simulink model "pdl_linear_hw4hybrid"  (R2017a)
settings: Solver=FixedStepAuto  StartTime=0.0  StopTime=duration  FixedStep=Ts  RelTol=1e-3
values from neighbouring files (symbols this model uses):
  A_a = [A E*Cw; zeros(2,4) Aw]    [pendulum_hw4linear.m]
  B_a = [B; zeros(2,1)]    [pendulum_hw4linear.m]
  C_a = [C zeros(2,2)]    [pendulum_hw4linear.m]
  E_a = [zeros(4,2); Bw]    [pendulum_hw4linear.m]
  f_p = 1e-4    (= 0.0001)    [pendulum_hw4linear.m]
  m_p = 1e-7    (= 1e-07)    [pendulum_hw4linear.m]
  Q_k1 = diag([10.00001 10.001])    [pendulum_hw4linear.m]
  Q_k2 = diag([10.00007 9.997])    [pendulum_hw4linear.m]
  Q_k3 = diag([10.0000905 9.995])    [pendulum_hw4linear.m]
  Q_k4 = diag([10.000101 9.9935])    [pendulum_hw4linear.m]
  R_k1 = 1e-5*diag([1 1])    [pendulum_hw4linear.m]
  R_k2 = 1e-5*diag([1 1])    [pendulum_hw4linear.m]
  R_k3 = 1e-5*diag([1 1])    [pendulum_hw4linear.m]
  R_k4 = 1e-5*diag([1 1])    [pendulum_hw4linear.m]
  Ts = 0.001    [pendulum_hw4linear.m]
  w_p = 10    [pendulum_hw4linear.m]
  X_0 = [0;0*pi/180;0;0;0;0]    [pendulum_hw4linear.m]
undefined symbols (not defined in the file or in its folder): Delta, Gamma, LC1_D, LC2_D, LC3_D, LC4_D, Phi
libraries: simulink x3
settings Model: Creator=Salmon  LastModifiedBy=Salmon

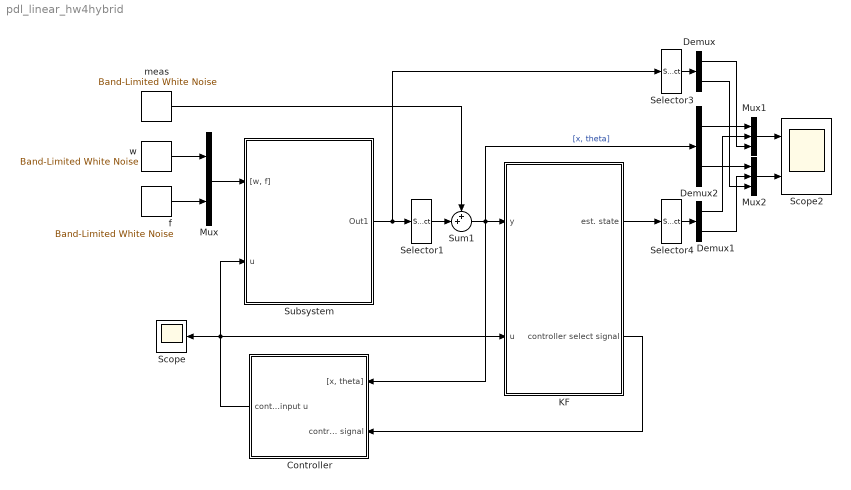
== system pdl_linear_hw4hybrid ==
  Controller : Subsystem
  Demux : Demux  Outputs=2
  Demux1 : Demux  Outputs=2
  Demux2 : Demux  Outputs=2
  KF : Subsystem
  Mux : Mux  Inputs=2
  Mux1 : Mux  Inputs=3
  Mux2 : Mux  Inputs=3
  Scope : Scope
  Scope2 : Scope  NumInputPorts=2
  Selector1 : Selector  InputPortWidth=6  IndexOptions=Index vector (dialog)  Indices=[1 2]  OutputSizes=1
  Selector3 : Selector  InputPortWidth=6  IndexOptions=Index vector (dialog)  Indices=[1 2]  OutputSizes=1
  Selector4 : Selector  InputPortWidth=6  IndexOptions=Index vector (dialog)  Indices=[1 2]  OutputSizes=1
  Subsystem : Subsystem
  Sum1 : Sum  Inputs=++|
  f : simulink/Sources/Band-Limited White Noise  Cov=[f_p]  Ts=Ts  seed=[23341]
  meas : simulink/Sources/Band-Limited White Noise  Cov=[m_p,m_p]  Ts=Ts  seed=[123,23341]
  w : simulink/Sources/Band-Limited White Noise  Cov=[w_p]  Ts=Ts  seed=[23341]
  wires:
  w/1 -> Mux/1
  f/1 -> Mux/2
  Mux/1 -> Subsystem/1("[w, f]")
  Subsystem/1(Out1) -> Selector1/1, Selector3/1
  Demux/1 -> Mux1/3
  Demux/2 -> Mux2/3
  Selector1/1 -> Sum1/2
  Demux1/1 -> Mux1/2
  KF/2(controller select signal) -> Controller/2(controller select signal)
  Demux1/2 -> Mux2/2
  meas/1 -> Sum1/1
  Demux2/1 -> Mux1/1
  Demux2/2 -> Mux2/1
  Mux1/1 -> Scope2/1
  Mux2/1 -> Scope2/2
  Sum1/1 -> Controller/1("[x, theta]"), KF/1(y), Demux2/1  "[x, theta]"
  Selector3/1 -> Demux/1
  Selector4/1 -> Demux1/1
  Controller/1(control input u) -> Subsystem/2(u), KF/2(u), Scope/1
  KF/1(est. state) -> Selector4/1

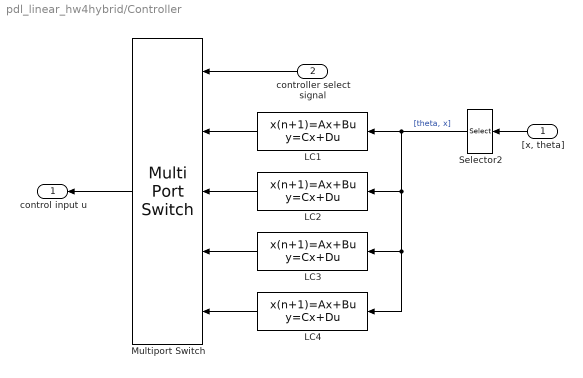
== system pdl_linear_hw4hybrid/Controller ==
  "[x, theta]" : Inport
  controller select signal : Inport  Port=2
  LC1 : DiscreteStateSpace  A=LC1_D.A  B=LC1_D.B  C=LC1_D.C  D=LC1_D.D  SampleTime=Ts
  LC2 : DiscreteStateSpace  A=LC2_D.A  B=LC2_D.B  C=LC2_D.C  D=LC2_D.D  SampleTime=Ts
  LC3 : DiscreteStateSpace  A=LC3_D.A  B=LC3_D.B  C=LC3_D.C  D=LC3_D.D  SampleTime=Ts
  LC4 : DiscreteStateSpace  A=LC4_D.A  B=LC4_D.B  C=LC4_D.C  D=LC4_D.D  SampleTime=Ts
  Multiport Switch : MultiPortSwitch  Inputs=4  DiagnosticForDefault=None
  Selector2 : Selector  InputPortWidth=2  IndexOptions=Index vector (dialog)  Indices=[2 1]  OutputSizes=1
  control input u : Outport
  wires:
  LC4/1 -> Multiport Switch/5
  controller select signal/1 -> Multiport Switch/1
  LC3/1 -> Multiport Switch/4
  LC2/1 -> Multiport Switch/3
  LC1/1 -> Multiport Switch/2
  Selector2/1 -> LC4/1, LC3/1, LC2/1, LC1/1  "[theta, x]"
  Multiport Switch/1 -> control input u/1
  "[x, theta]"/1 -> Selector2/1

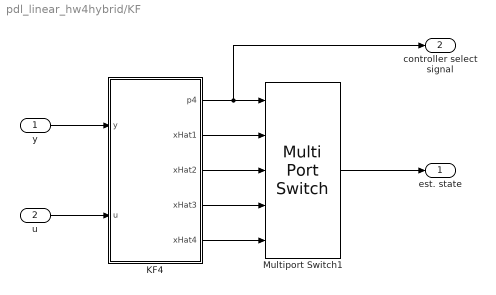
== system pdl_linear_hw4hybrid/KF ==
  y : Inport
  u : Inport  Port=2
  KF4 : Subsystem
  Multiport Switch1 : MultiPortSwitch  Inputs=4  DiagnosticForDefault=None
  est. state : Outport
  controller select signal : Outport  Port=2
  wires:
  u/1 -> KF4/2(u)
  Multiport Switch1/1 -> est. state/1
  y/1 -> KF4/1(y)
  KF4/5("xHat4 ") -> Multiport Switch1/5
  KF4/4(xHat3) -> Multiport Switch1/4
  KF4/3(xHat2) -> Multiport Switch1/3
  KF4/2(xHat1) -> Multiport Switch1/2
  KF4/1(p4) -> controller select signal/1, Multiport Switch1/1

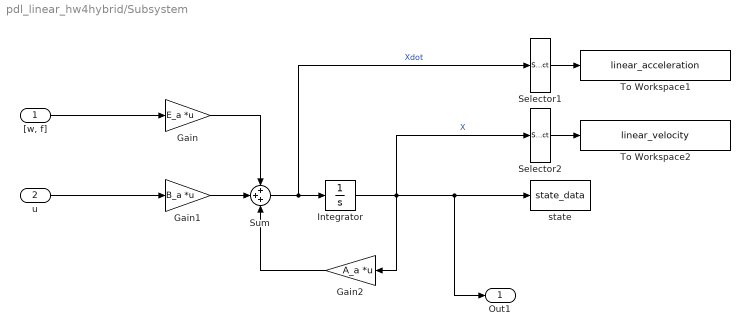
== system pdl_linear_hw4hybrid/Subsystem ==
  "[w, f]" : Inport
  u : Inport  Port=2
  Gain : Gain  Gain=E_a  Multiplication=Matrix(K*u)
  Gain1 : Gain  Gain=B_a  Multiplication=Matrix(K*u)
  Gain2 : Gain  Gain=A_a  Multiplication=Matrix(K*u)
  Integrator : Integrator  InitialCondition=X_0
  Selector1 : Selector  InputPortWidth=6  IndexOptions=Index vector (dialog)  Indices=[3]  OutputSizes=1
  Selector2 : Selector  InputPortWidth=6  IndexOptions=Index vector (dialog)  Indices=[3]  OutputSizes=1
  Sum : Sum  Inputs=+++
  To Workspace1 : ToWorkspace  VariableName=linear_acceleration  SaveFormat=Structure With Time  SampleTime=-1
  To Workspace2 : ToWorkspace  VariableName=linear_velocity  SaveFormat=Structure With Time  SampleTime=-1
  state : ToWorkspace  VariableName=state_data  SaveFormat=Structure With Time  SampleTime=Ts
  Out1 : Outport
  wires:
  "[w, f]"/1 -> Gain/1
  Gain/1 -> Sum/1
  Gain1/1 -> Sum/2
  Selector2/1 -> To Workspace2/1
  Selector1/1 -> To Workspace1/1
  Gain2/1 -> Sum/3
  u/1 -> Gain1/1
  Integrator/1 -> Gain2/1, Selector2/1, Out1/1, state/1  "X"
  Sum/1 -> Integrator/1, Selector1/1  "Xdot"

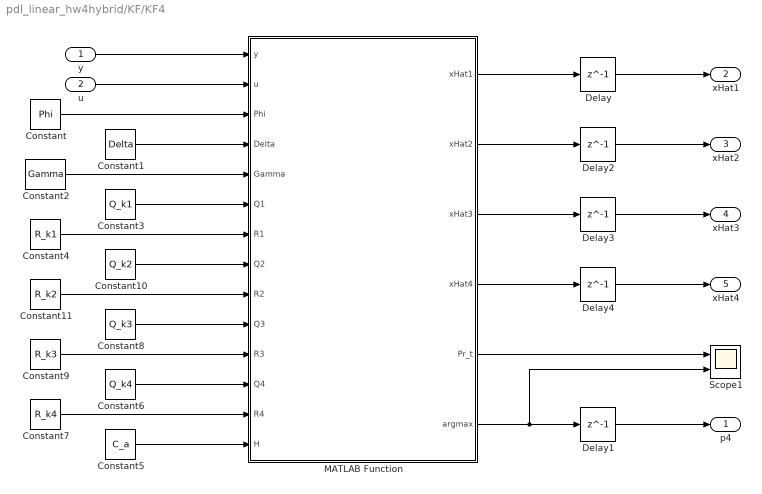
== system pdl_linear_hw4hybrid/KF/KF4 ==
  y : Inport
  u : Inport  Port=2
  Constant : Constant  Value=Phi
  Constant1 : Constant  Value=Delta
  Constant10 : Constant  Value=Q_k2
  Constant11 : Constant  Value=R_k2
  Constant2 : Constant  Value=Gamma
  Constant3 : Constant  Value=Q_k1
  Constant4 : Constant  Value=R_k1
  Constant5 : Constant  Value=C_a
  Constant6 : Constant  Value=Q_k4
  Constant7 : Constant  Value=R_k4
  Constant8 : Constant  Value=Q_k3
  Constant9 : Constant  Value=R_k3
  Delay{,1..4} (5 alike) : Delay  DelayLength=1  InitialCondition=0
  MATLAB Function : MATLAB Function  TreatAsAtomicUnit=on
  Scope1 : Scope  NumInputPorts=2
  p4 : Outport
  xHat1 : Outport  Port=2
  xHat2 : Outport  Port=3
  xHat3 : Outport  Port=4
  "xHat4 " : Outport  Port=5
  wires:
  Constant3/1 -> MATLAB Function/6(Q1)
  MATLAB Function/1(xHat1) -> Delay/1
  Constant5/1 -> MATLAB Function/14(H)
  Delay/1 -> xHat1/1
  Constant1/1 -> MATLAB Function/4(Delta)
  Constant/1 -> MATLAB Function/3(Phi)
  Constant4/1 -> MATLAB Function/7(R1)
  Constant2/1 -> MATLAB Function/5(Gamma)
  u/1 -> MATLAB Function/2(u)
  y/1 -> MATLAB Function/1(y)
  Delay1/1 -> p4/1
  MATLAB Function/6(argmax) -> Scope1/2, Delay1/1
  Constant6/1 -> MATLAB Function/12(Q4)
  Constant7/1 -> MATLAB Function/13(R4)
  Constant8/1 -> MATLAB Function/10(Q3)
  Constant9/1 -> MATLAB Function/11(R3)
  Constant10/1 -> MATLAB Function/8(Q2)
  Constant11/1 -> MATLAB Function/9(R2)
  MATLAB Function/2(xHat2) -> Delay2/1
  Delay2/1 -> xHat2/1
  MATLAB Function/3(xHat3) -> Delay3/1
  Delay3/1 -> xHat3/1
  MATLAB Function/4(xHat4) -> Delay4/1
  Delay4/1 -> "xHat4 "/1
  MATLAB Function/5(Pr_t) -> Scope1/1

== matlab function pdl_linear_hw4hybrid/KF/KF4/MATLAB Function ==
  data: y input; u input; xHat1 output; xHat2 output; xHat3 output; xHat4 output; Pr_t output; Phi input; Delta input; Gamma input; Q1 input; R1 input; Q2 input; R2 input; Q3 input; R3 input; Q4 input; R4 input; H input; argmax output
function [xHat1,xHat2,xHat3,xHat4,Pr_t,argmax] = fcn(y,u,Phi,Delta,Gamma,Q1,R1,Q2,R2,Q3,R3,Q4,R4,H)

%persistent Pbar 
persistent xbar1 Sig1 Pr1 
persistent xbar2 Sig2 Pr2
persistent xbar3 Sig3 Pr3
persistent xbar4 Sig4 Pr4

if isempty(xbar1) xbar1 = zeros(6,1);  end

if isempty(Sig1)  Sig1 = 1e-4*eye(6);  end

if isempty(Pr1)   Pr1 = 0.25*eye(2);   end

if isempty(xbar2) xbar2 = zeros(6,1);  end

if isempty(Sig2)  Sig2 = 1e-4*eye(6);  end

if isempty(Pr2)   Pr2 = 0.25*eye(2);   end

if isempty(xbar3) xbar3 = zeros(6,1);  end

if isempty(Sig3)  Sig3 = 1e-4*eye(6);  end

if isempty(Pr3)   Pr3 = 0.25*eye(2);   end

if isempty(xbar4) xbar4 = zeros(6,1);  end

if isempty(Sig4)  Sig4 = 1e-4*eye(6);  end

if isempty(Pr4)   Pr4 = 0.25*eye(2);   end

% KF1
K_hi1 = Sig1*H'*(H*Sig1*H'+R1)^(-1);
y_o1 = H*xbar1;
y_e1 = y-y_o1;
Sig_hat1 = (eye(6)-K_hi1*H)*Sig1*(eye(6)-K_hi1*H)'+K_hi1*R1*K_hi1';
xHat1 = xbar1 + K_hi1*y_e1;
xbar1 = Phi*xHat1+Delta*u;
Sig1 = Phi*Sig_hat1*Phi'+Gamma*Q1*Gamma';
S_hi1 = H*Sig1*H' + R1;

Pr_numerator1 = exp(-0.5*y_e1'*S_hi1^(-1)*y_e1)*Pr1*(sqrt((2*pi)^3*abs(S_hi1)))^(-1);

% KF2
K_hi2 = Sig2*H'*(H*Sig2*H'+R2)^(-1);
y_o2 = H*xbar2;
y_e2 = y-y_o2;
Sig_hat2 = (eye(6)-K_hi2*H)*Sig2*(eye(6)-K_hi2*H)'+K_hi2*R2*K_hi2';
xHat2 = xbar2 + K_hi2*y_e2;
xbar2 = Phi*xHat2+Delta*u;
Sig2 = Phi*Sig_hat2*Phi'+Gamma*Q2*Gamma';
S_hi2 = H*Sig2*H' + R2;

Pr_numerator2 = exp(-0.5*y_e2'*S_hi2^(-1)*y_e2)*Pr2*(sqrt((2*pi)^3*abs(S_hi2)))^(-1);

% KF3
K_hi3 = Sig3*H'*(H*Sig3*H'+R3)^(-1);
y_o3 = H*xbar3;
y_e3 = y-y_o3;
Sig_hat3 = (eye(6)-K_hi3*H)*Sig3*(eye(6)-K_hi3*H)'+K_hi3*R3*K_hi3';
xHat3 = xbar3 + K_hi3*y_e3;
xbar3 = Phi*xHat3+Delta*u;
Sig3 = Phi*Sig_hat3*Phi'+Gamma*Q3*Gamma';
S_hi3 = H*Sig3*H' + R3;

Pr_numerator3 = exp(-0.5*y_e3'*S_hi3^(-1)*y_e3)*Pr3*(sqrt((2*pi)^3*abs(S_hi3)))^(-1);

% KF4
K_hi4 = Sig4*H'*(H*Sig4*H'+R4)^(-1);
y_o4 = H*xbar4;
y_e4 = y-y_o4;
Sig_hat4 = (eye(6)-K_hi4*H)*Sig4*(eye(6)-K_hi4*H)'+K_hi4*R4*K_hi4';
xHat4 = xbar4 + K_hi4*y_e4;
xbar4 = Phi*xHat4+Delta*u;
Sig4 = Phi*Sig_hat4*Phi'+Gamma*Q4*Gamma';
S_hi4 = H*Sig4*H' + R4;

% Calculate conditional probabilities
Pr_numerator4 = exp(-0.5*y_e4'*S_hi4^(-1)*y_e4)*Pr4*(sqrt((2*pi)^3*abs(S_hi4)))^(-1);

Pr_denom = Pr_numerator1 + Pr_numerator2 + Pr_numerator3 + Pr_numerator4;
Pr1 = Pr_numerator1/Pr_denom;
Pr2 = Pr_numerator2/Pr_denom;
Pr3 = Pr_numerator3/Pr_denom;
Pr4 = Pr_numerator4/Pr_denom;

Pr_t = [Pr1(1,1),Pr2(1,1),Pr3(1,1),Pr4(1,1)];

% Maximum likelihood
[~,argmax] = max(Pr_t);
